simulink model "TwoLinkRobotNLEx"  (R2018b)
settings: Solver=VariableStepAuto  StartTime=0.0  StopTime=5  RelTol=1e-3
values from neighbouring files (symbols this model uses):
  KSfb = -Klqr    [twoLinkRobot_powerit.m]
undefined symbols (not defined in the file or in its folder): alpha, beta, delta, eta0
libraries: ltvlib x3
settings Model: Creator=pjseiler  LastModifiedBy=Jyot Buch
settings DataIOCC: ExternalInput=simInput
settings SFSimCC: SimUseLocalCustomCode=off
settings RTWCC: RTWUseLocalCustomCode=off
settings CodeAppCC: StateflowObjectComments=on

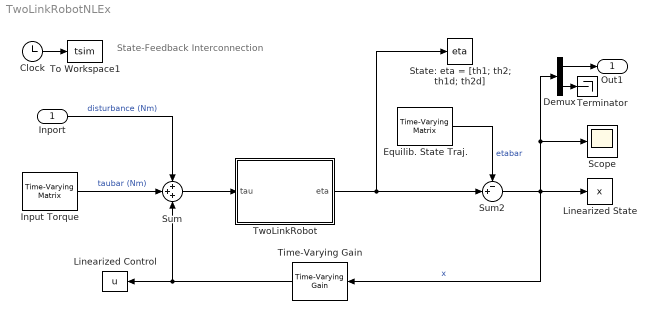
== system TwoLinkRobotNLEx ==
  note: State-Feedback Interconnection
  Inport : Inport  PortDimensions=2
  Clock : Clock
  Demux : Demux  Outputs=[2;2]
  Equilib. State Traj. : ltvlib/Time-Varying Matrix  M=etabar  vec1D=on
      settings: SourceProductName=Linear Time-Varying Systems Toolbox
  Input Torque : ltvlib/Time-Varying Matrix  M=taubar  vec1D=on
      settings: SourceProductName=Linear Time-Varying Systems Toolbox
  Linearized Control : ToWorkspace  VariableName=u  SampleTime=-1
  Linearized State : ToWorkspace  VariableName=x  SampleTime=-1
  Scope : Scope
  State: eta = [th1; th2; th1d; th2d] : ToWorkspace  VariableName=eta  SampleTime=-1
  Sum : Sum  Inputs=+++
  Sum2 : Sum  Inputs=-+|
  Terminator : Terminator
  Time-Varying Gain : ltvlib/Time-Varying Gain  K=KSfb
      settings: SourceProductName=Linear Time-Varying Systems Toolbox
  To Workspace1 : ToWorkspace  VariableName=tsim  SampleTime=-1
  TwoLinkRobot : Subsystem
  Out1 : Outport
  wires:
  Clock/1 -> To Workspace1/1
  Inport/1 -> Sum/1  "disturbance (Nm)"
  TwoLinkRobot/1(eta) -> State: eta = [th1; th2; th1d; th2d]/1, Sum2/2
  Equilib. State Traj./1 -> Sum2/1  "etabar"
  Sum2/1 -> Time-Varying Gain/1, Demux/1, Scope/1, Linearized State/1  "x"
  Time-Varying Gain/1 -> Linearized Control/1, Sum/3
  Input Torque/1 -> Sum/2  "taubar (Nm)"
  Sum/1 -> TwoLinkRobot/1(tau)
  Demux/2 -> Terminator/1
  Demux/1 -> Out1/1

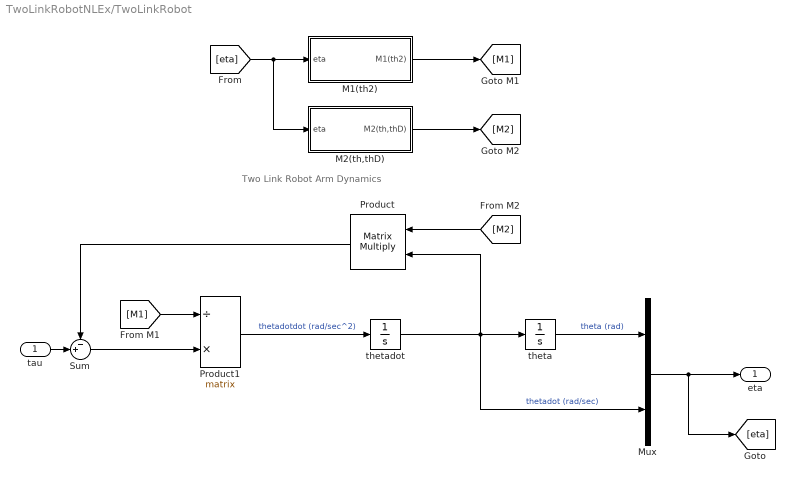
== system TwoLinkRobotNLEx/TwoLinkRobot ==
  note: Two Link Robot Arm Dynamics
  tau : Inport  PortDimensions=2
  M1(th2) : Subsystem  TreatAsAtomicUnit=on
  M2(th,thD) : Subsystem  TreatAsAtomicUnit=on
  Mux : Mux  Inputs=2
  Product : Product  Inputs=**  Multiplication=Matrix(*)
  Product1 : Product  Inputs=/*  Multiplication=Matrix(*)
  Sum : Sum  Inputs=-+|
  theta : Integrator  InitialCondition=eta0(1:2)
  thetadot : Integrator  InitialCondition=eta0(3:4)
  eta : Outport
  wires:
  M1(th2)/1(M1(th2)) -> [M1]
  Product1/1 -> thetadot/1  "thetadotdot (rad/sec^2)"
  Mux/1 -> [eta], eta/1
  [eta] -> M2(th,thD)/1(eta), M1(th2)/1(eta)
  thetadot/1 -> Mux/2, Product/2, theta/1  "thetadot (rad/sec)"
  M2(th,thD)/1(M2(th,thD)) -> [M2]
  Product/1 -> Sum/1
  Sum/1 -> Product1/2
  [M1] -> Product1/1
  tau/1 -> Sum/2
  [M2] -> Product/1
  theta/1 -> Mux/1  "theta (rad)"

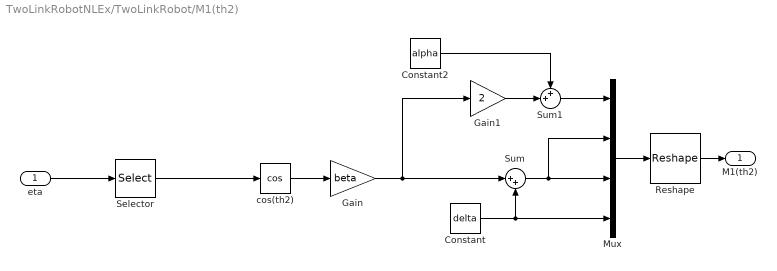
== system TwoLinkRobotNLEx/TwoLinkRobot/M1(th2) ==
  eta : Inport
  Constant : Constant  Value=delta
  Constant2 : Constant  Value=alpha
  Gain : Gain  Gain=beta
  Gain1 : Gain  Gain=2
  Mux : Mux
  Reshape : Reshape  OutputDimensionality=Customize  OutputDimensions=[2 2]
  Selector : Selector  InputPortWidth=4  IndexOptions=Index vector (dialog)  Indices=2  OutputSizes=1
  Sum : Sum  Inputs=|++
  Sum1 : Sum  Inputs=++|
  cos(th2) : Trigonometry  Operator=cos
  M1(th2) : Outport
  wires:
  Reshape/1 -> M1(th2)/1
  Mux/1 -> Reshape/1
  Constant/1 -> Mux/4, Sum/2
  Sum/1 -> Mux/3, Mux/2
  cos(th2)/1 -> Gain/1
  Gain/1 -> Gain1/1, Sum/1
  Constant2/1 -> Sum1/1
  Sum1/1 -> Mux/1
  Gain1/1 -> Sum1/2
  eta/1 -> Selector/1
  Selector/1 -> cos(th2)/1

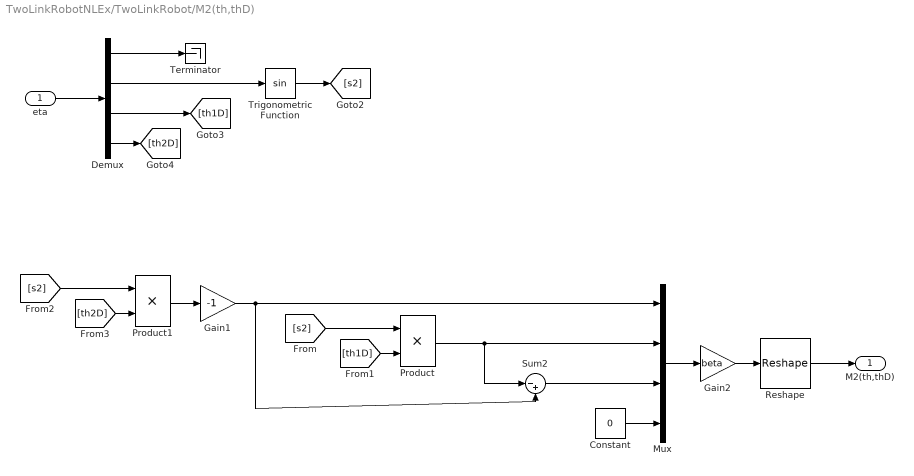
== system TwoLinkRobotNLEx/TwoLinkRobot/M2(th,thD) ==
  eta : Inport
  Constant : Constant  Value=0
  Demux : Demux
  Gain1 : Gain  Gain=-1
  Gain2 : Gain  Gain=beta
  Mux : Mux
  Product : Product
  Product1 : Product
  Reshape : Reshape  OutputDimensionality=Customize  OutputDimensions=[2 2]
  Sum2 : Sum  Inputs=|-+
  Terminator : Terminator
  Trigonometric Function : Trigonometry
  M2(th,thD) : Outport
  wires:
  Constant/1 -> Mux/4
  Reshape/1 -> M2(th,thD)/1
  eta/1 -> Demux/1
  Demux/4 -> [th2D]
  Demux/1 -> Terminator/1
  Demux/2 -> Trigonometric Function/1
  Demux/3 -> [th1D]
  Trigonometric Function/1 -> [s2]
  [s2] -> Product/1
  [th1D] -> Product/2
  Product/1 -> Sum2/1, Mux/2
  Gain2/1 -> Reshape/1
  Mux/1 -> Gain2/1
  [th2D] -> Product1/2
  [s2] -> Product1/1
  Product1/1 -> Gain1/1
  Sum2/1 -> Mux/3
  Gain1/1 -> Sum2/2, Mux/1
